simulink library "sltestHeatpumpLibraryExample"  (R2017a)
settings: Solver=VariableStepAuto  StartTime=0.0  StopTime=10.0  RelTol=1e-3  EnableMultiTasking=on
PostLoadFcn:
  | load 'sltestHeatpumpBusPostLoadFcn.mat'
libraries: simulink x1
settings Model: Creator=The MathWorks, Inc.  LastModifiedBy=The MathWorks, Inc.
settings DataIOCC: LimitDataPoints=on
settings OptimizationCC: LifeSpan=inf
settings DebuggingCC: AllowSymbolicDim=off  SFUnexpectedBacktrackingDiag=warning  SFNoUnconditionalDefaultTransitionDiag=warning  SFExecutionAtInitializationDiag=none
settings ModelReferenceCC: PropagateSignalLabelsOutOfModel=off
settings GRTTargetCC: TargetLangStandard=C89/C90 (ANSI)
settings ConfigComp: CovMetricSettings=dw  CovHtmlReporting=on  CovSaveCumulativeToWorkspaceVar=on  CovSaveSingleToWorkspaceVar=on  CovExternalEMLEnable=off

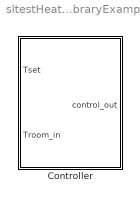
== system sltestHeatpumpLibraryExample ==
  Controller : Subsystem  TreatAsAtomicUnit=on  SystemSampleTime=1

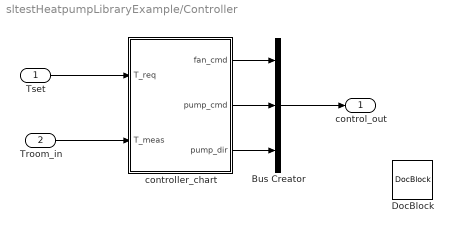
== system sltestHeatpumpLibraryExample/Controller ==
  Tset : Inport
  Troom_in : Inport  Port=2
  Bus Creator : BusCreator  Inputs=3  OutDataTypeStr=Bus: control_bus  NonVirtualBus=on
  DocBlock : simulink/Model-Wide Utilities/DocBlock  DocumentType=Text
      content=|
      | Requirements for the basic Heatpump Controller
      |
      | Temperature difference is defined as the difference between the room and
      | the set temperature.  The controller shall turn the fan on when the
      | temperature difference has reached a certain level, to circulate the air.
      | The controller shall turn the heatpump on when the temperature difference
      | has reached another level, to heat or cool the space.
      |
      | 1. If the temperature difference is less than 2 degrees, the system shall
      | be idle with all signals off.
      | 2. The fan shall activate when the temperature difference is greater than
      | or equal to 2 degrees.
      | 3. The pump shall activate when the temperature difference is greater than
      | or equal to 4 degrees.
      |     3a. If the room temperature is greater than the set temperature, the
      |         system shall cool the space.
      |     3b. If the room temperature is less than the set temperature, the system
      |         shall heat the space.
  controller_chart : Stateflow chart  TreatAsAtomicUnit=on
  control_out : Outport
  wires:
  controller_chart/2(pump_cmd) -> Bus Creator/2
  controller_chart/1(fan_cmd) -> Bus Creator/1
  controller_chart/3(pump_dir) -> Bus Creator/3
  Bus Creator/1 -> control_out/1
  Tset/1 -> controller_chart/1(T_req)
  Troom_in/1 -> controller_chart/2(T_meas)

== stateflow chart sltestHeatpumpLibraryExample/Controller/controller_chart ==
  state IDLE
    entry:
    fan_cmd = 0;
    pump_cmd = 0;
    pump_dir = 0;
  state RUNNING
    state FAN_ONLY
      entry:
      fan_cmd = 1;
      pump_cmd = 0;
      pump_dir = 0;
    state COOLING
      entry:
      fan_cmd = 1;
      pump_cmd = 1;
      pump_dir = 1;
    state HEATING
      entry:
      fan_cmd = 1;
      pump_cmd = 1;
      pump_dir = -1;
    (default) -> FAN_ONLY
    HEATING -> FAN_ONLY : after(2,sec)
        | [mag_T(T_req,T_meas) < 4]
    COOLING -> FAN_ONLY : after(2,sec)
        | [mag_T(T_req,T_meas) < 4]
    FAN_ONLY -> (junction 49) : after(2,sec)
        | [mag_T(T_req,T_meas) >= 4]
    (junction 49) -> COOLING [order 1] : [sign_T(T_req, T_meas) == -1]
    (junction 49) -> HEATING [order 2]
  (default) -> IDLE
  RUNNING -> IDLE : [mag_T(T_req,T_meas) < 2]
  IDLE -> RUNNING : [mag_T(T_req,T_meas) >= 2]
  data: T_req_in function_input double size=1; T_meas_in function_input double size=1; Mag function_output double size=1; T_req_in function_input double size=1; T_meas_in function_input double size=1; Tdir function_output double size=1; fan_cmd output boolean =false; pump_cmd output boolean =false; pump_dir output int16 [-1..1] =0; T_req input double size=1; T_meas input double size=1
  function Mag  = mag_T(T_req_in, T_meas_in):
    | function Mag  = mag_T(T_req_in, T_meas_in)
    | %#codegen
    | 
    | Mag = abs(T_req_in - T_meas_in);
  function Tdir = sign_T(T_req_in,T_meas_in):
    | function Tdir = sign_T(T_req_in,T_meas_in)
    |  %#codegen
    |  
    | Tdir = sign(T_req_in - T_meas_in);
